simulink model "TVC_3D"  (R2020b)
settings: Solver=VariableStepAuto  StartTime=0.0  StopTime=10.0  RelTol=1e-3
libraries: pid_lib x2, shared6dof x1
settings Model: Creator=mluser  LastModifiedBy=avina

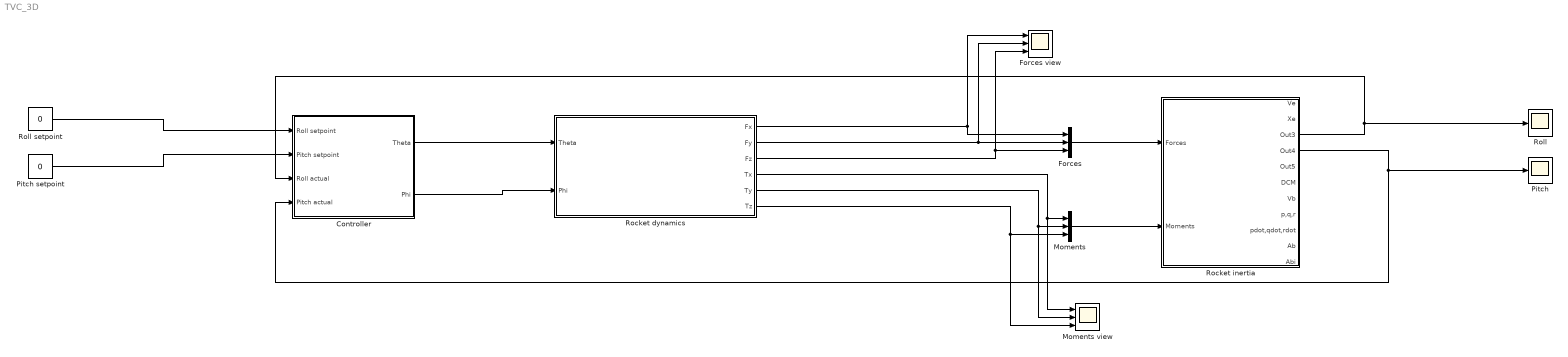
== system TVC_3D ==
  Controller : Subsystem
  Forces : Mux  Inputs=3
  Forces view : Scope  NumInputPorts=3
  Moments : Mux  Inputs=3
  Moments view : Scope  NumInputPorts=3
  Pitch : Scope
  Pitch setpoint : Constant  Value=0
  Rocket dynamics : Subsystem
  Rocket inertia : Subsystem
  Roll : Scope
  Roll setpoint : Constant  Value=0
  wires:
  Roll setpoint/1 -> Controller/1(Roll setpoint)
  Pitch setpoint/1 -> Controller/2(Pitch setpoint)
  Rocket dynamics/4(Tx) -> Moments view/1, Moments/1
  Rocket dynamics/3(Fz) -> Forces/3, Forces view/3
  Rocket dynamics/5(Ty) -> Moments view/2, Moments/2
  Rocket dynamics/1(Fx) -> Forces view/1, Forces/1
  Rocket dynamics/2(Fy) -> Forces view/2, Forces/2
  Rocket dynamics/6(Tz) -> Moments view/3, Moments/3
  Controller/1(Theta) -> Rocket dynamics/1(Theta)
  Controller/2(Phi) -> Rocket dynamics/2(Phi)
  Rocket inertia/4(Out4) -> Controller/4(Pitch actual), Pitch/1
  Rocket inertia/3(Out3) -> Controller/3(Roll actual), Roll/1
  Forces/1 -> Rocket inertia/1(Forces)
  Moments/1 -> Rocket inertia/2(Moments)

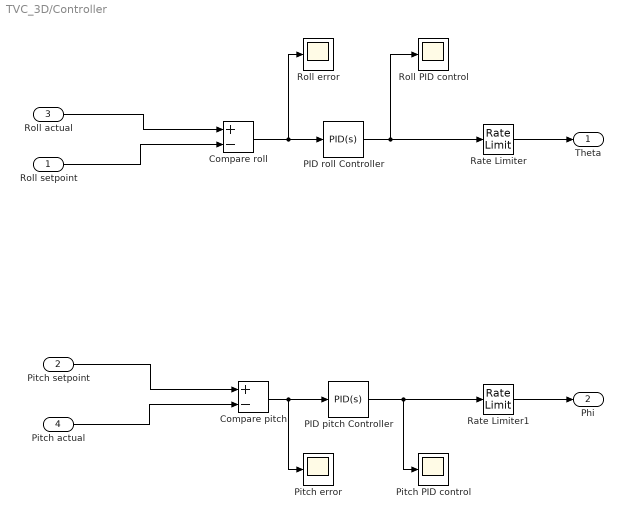
== system TVC_3D/Controller ==
  Roll setpoint : Inport
  Pitch setpoint : Inport  Port=2
  Roll actual : Inport  Port=3
  Pitch actual : Inport  Port=4
  Compare pitch : Sum  Inputs=+-
  Compare roll : Sum  Inputs=+-
  PID pitch Controller : pid_lib/PID Controller  Controller=PID  Form=Parallel  TimeDomain=Continuous-time  UseExternalTs=off  SampleTime=-1  IntegratorMethod=Forward Euler  FilterMethod=Forward Euler  ControllerParametersSource=internal  P=0.2  I=0.00047  D=0.06  UseFilter=on  N=100  TunerSelectOption=Transfer Function Based (PID Tuner App)  InitialConditionSource=internal  InitialConditionForIntegrator=0  InitialConditionForFilter=0  DifferentiatorICPrevScaledInput=0  ExternalReset=none  TrackingMode=off  Kt=1  LimitOutput=on  SatLimitsSource=internal  UpperSaturationLimit=0.349  LowerSaturationLimit=-0.349  LinearizeAsGain=on  AntiWindupMode=none  Kb=1  POutMin=[]  POutMax=[]  IOutMin=[]  IOutMax=[]  DOutMin=[]  DOutMax=[]  NOutMin=[]  NOutMax=[]  SumOutMin=[]  SumOutMax=[]  SaturationOutMin=[]  SaturationOutMax=[]  PParamMin=[]  PParamMax=[]  IParamMin=[]  IParamMax=[]  DParamMin=[]  DParamMax=[]  NParamMin=[]  NParamMax=[]  KbParamMin=[]  KbParamMax=[]  KtParamMin=[]  KtParamMax=[]  KbOutMin=[]  KbOutMax=[]  KtOutMin=[]  KtOutMax=[]  IntegratorOutMin=[]  IntegratorOutMax=[]  FilterOutMin=[]  FilterOutMax=[]  SumI1OutMin=[]  SumI1OutMax=[]  SumI2OutMin=[]  SumI2OutMax=[]  SumI3OutMin=[]  SumI3OutMax=[]  SumI4OutMin=[]  SumI4OutMax=[]  SumDOutMin=[]  SumDOutMax=[]  DifferentiatorOutMin=[]  DifferentiatorOutMax=[]  FilterDiffOutCoefMin=[]  FilterDiffOutCoefMax=[]  ReciprocalOutMin=[]  ReciprocalOutMax=[]  SumDenOutMin=[]  SumDenOutMax=[]  SumNumOutMin=[]  SumNumOutMax=[]  DivideOutMin=[]  DivideOutMax=[]  UdiffTsProdOutMin=[]  UdiffTsProdOutMax=[]  NTsProdOutMin=[]  NTsProdOutMax=[]  UintegralTsProdOutMin=[]  UintegralTsProdOutMax=[]  UngainTsProdOutMin=[]  UngainTsProdOutMax=[]  IntegratorContinuousStateAttributes=''  IntegratorStateMustResolveToSignalObject=off  IntegratorRTWStateStorageClass=Auto  FilterContinuousStateAttributes=''  FilterStateMustResolveToSignalObject=off  FilterRTWStateStorageClass=Auto  ParallelPVariant=InternalParameters  IdealPVariant=Disabled  IVariant=InternalParameters  DVariant=InternalParameters  IntegratorVariant=Continuous  SatVariant=Enabled  AWVariant=Passthrough  PCopyVariant=Disabled  TRVariant=Disabled  FdbkBlocksVariant=Forward  IdealPFdbkVariant=Disabled  SatFdbkVariant=Disabled  DerivativeFilterVariant=ContFilter  NVariant=InternalParameters  NCopyVariant=Disabled  FilterICVariant=InternalICsFilter  IntegratorICVariant=InternalICs  ExternalResetVariant=Disabled  TRSumVariant=Passthrough  SumFdbkVariant=Disabled  SumVariant=Sum_PID  TsampFilterVariant=InternalTs  TsampNgainVariant=Passthrough  TsampIntegralVariant=Passthrough  ExternalSaturationOutDataTypeStr=Inherit: Same as second input
  PID roll Controller : pid_lib/PID Controller  Controller=PID  Form=Parallel  TimeDomain=Continuous-time  UseExternalTs=off  SampleTime=-1  IntegratorMethod=Forward Euler  FilterMethod=Forward Euler  ControllerParametersSource=internal  P=0.2  I=0  D=0.06  UseFilter=on  N=100  TunerSelectOption=Transfer Function Based (PID Tuner App)  InitialConditionSource=internal  InitialConditionForIntegrator=0  InitialConditionForFilter=0  DifferentiatorICPrevScaledInput=0  ExternalReset=none  TrackingMode=off  Kt=1  LimitOutput=on  SatLimitsSource=internal  UpperSaturationLimit=0.349  LowerSaturationLimit=-0.349  LinearizeAsGain=on  AntiWindupMode=none  Kb=1  POutMin=[]  POutMax=[]  IOutMin=[]  IOutMax=[]  DOutMin=[]  DOutMax=[]  NOutMin=[]  NOutMax=[]  SumOutMin=[]  SumOutMax=[]  SaturationOutMin=[]  SaturationOutMax=[]  PParamMin=[]  PParamMax=[]  IParamMin=[]  IParamMax=[]  DParamMin=[]  DParamMax=[]  NParamMin=[]  NParamMax=[]  KbParamMin=[]  KbParamMax=[]  KtParamMin=[]  KtParamMax=[]  KbOutMin=[]  KbOutMax=[]  KtOutMin=[]  KtOutMax=[]  IntegratorOutMin=[]  IntegratorOutMax=[]  FilterOutMin=[]  FilterOutMax=[]  SumI1OutMin=[]  SumI1OutMax=[]  SumI2OutMin=[]  SumI2OutMax=[]  SumI3OutMin=[]  SumI3OutMax=[]  SumI4OutMin=[]  SumI4OutMax=[]  SumDOutMin=[]  SumDOutMax=[]  DifferentiatorOutMin=[]  DifferentiatorOutMax=[]  FilterDiffOutCoefMin=[]  FilterDiffOutCoefMax=[]  ReciprocalOutMin=[]  ReciprocalOutMax=[]  SumDenOutMin=[]  SumDenOutMax=[]  SumNumOutMin=[]  SumNumOutMax=[]  DivideOutMin=[]  DivideOutMax=[]  UdiffTsProdOutMin=[]  UdiffTsProdOutMax=[]  NTsProdOutMin=[]  NTsProdOutMax=[]  UintegralTsProdOutMin=[]  UintegralTsProdOutMax=[]  UngainTsProdOutMin=[]  UngainTsProdOutMax=[]  IntegratorContinuousStateAttributes=''  IntegratorStateMustResolveToSignalObject=off  IntegratorRTWStateStorageClass=Auto  FilterContinuousStateAttributes=''  FilterStateMustResolveToSignalObject=off  FilterRTWStateStorageClass=Auto  ParallelPVariant=InternalParameters  IdealPVariant=Disabled  IVariant=InternalParameters  DVariant=InternalParameters  IntegratorVariant=Continuous  SatVariant=Enabled  AWVariant=Passthrough  PCopyVariant=Disabled  TRVariant=Disabled  FdbkBlocksVariant=Forward  IdealPFdbkVariant=Disabled  SatFdbkVariant=Disabled  DerivativeFilterVariant=ContFilter  NVariant=InternalParameters  NCopyVariant=Disabled  FilterICVariant=InternalICsFilter  IntegratorICVariant=InternalICs  ExternalResetVariant=Disabled  TRSumVariant=Passthrough  SumFdbkVariant=Disabled  SumVariant=Sum_PID  TsampFilterVariant=InternalTs  TsampNgainVariant=Passthrough  TsampIntegralVariant=Passthrough  ExternalSaturationOutDataTypeStr=Inherit: Same as second input
  Pitch PID control : Scope
  Pitch error : Scope
  Rate Limiter : RateLimiter  RisingSlewLimit=500  FallingSlewLimit=-500  SampleTimeMode=inherited
  Rate Limiter1 : RateLimiter  RisingSlewLimit=500  FallingSlewLimit=-500  SampleTimeMode=inherited
  Roll PID control : Scope
  Roll error : Scope
  Theta : Outport
  Phi : Outport  Port=2
  wires:
  PID pitch Controller/1 -> Pitch PID control/1, Rate Limiter1/1
  PID roll Controller/1 -> Roll PID control/1, Rate Limiter/1
  Roll setpoint/1 -> Compare roll/2
  Compare roll/1 -> Roll error/1, PID roll Controller/1
  Pitch actual/1 -> Compare pitch/2
  Compare pitch/1 -> Pitch error/1, PID pitch Controller/1
  Roll actual/1 -> Compare roll/1
  Pitch setpoint/1 -> Compare pitch/1
  Rate Limiter/1 -> Theta/1
  Rate Limiter1/1 -> Phi/1

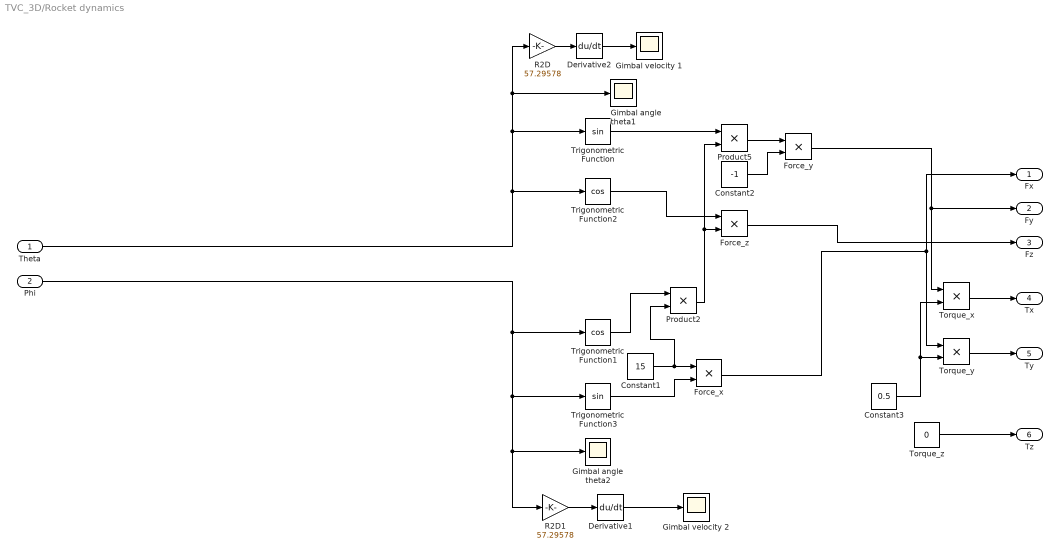
== system TVC_3D/Rocket dynamics ==
  Theta : Inport
  Phi : Inport  Port=2
  Constant1 : Constant  Value=15
  Constant2 : Constant  Value=-1
  Constant3 : Constant  Value=0.5
  Derivative1 : Derivative
  Derivative2 : Derivative
  Force_x : Product
  Force_y : Product
  Force_z : Product
  Gimbal angle theta1 : Scope
  Gimbal angle theta2 : Scope
  Gimbal velocity 1 : Scope
  Gimbal velocity 2 : Scope
  Product2 : Product
  Product5 : Product
  R2D : Gain  Gain=57.29578
  R2D1 : Gain  Gain=57.29578
  Torque_x : Product
  Torque_y : Product
  Torque_z : Constant  Value=0
  Trigonometric Function : Trigonometry
  Trigonometric Function1 : Trigonometry  Operator=cos
  Trigonometric Function2 : Trigonometry  Operator=cos
  Trigonometric Function3 : Trigonometry
  Fx : Outport
  Fy : Outport  Port=2
  Fz : Outport  Port=3
  Tx : Outport  Port=4
  Ty : Outport  Port=5
  Tz : Outport  Port=6
  wires:
  Product2/1 -> Product5/2, Force_z/2
  Derivative2/1 -> Gimbal velocity 1/1
  Theta/1 -> R2D/1, Gimbal angle theta1/1, Trigonometric Function/1, Trigonometric Function2/1
  Force_x/1 -> Fx/1, Torque_y/1
  Constant1/1 -> Force_x/1, Product2/2
  Trigonometric Function2/1 -> Force_z/1
  Phi/1 -> R2D1/1, Gimbal angle theta2/1, Trigonometric Function3/1, Trigonometric Function1/1
  Torque_x/1 -> Tx/1
  Torque_y/1 -> Ty/1
  Trigonometric Function3/1 -> Force_x/2
  Constant3/1 -> Torque_x/2, Torque_y/2
  Force_z/1 -> Fz/1
  Trigonometric Function/1 -> Product5/1
  Product5/1 -> Force_y/1
  Constant2/1 -> Force_y/2
  Trigonometric Function1/1 -> Product2/1
  Force_y/1 -> Torque_x/1, Fy/1
  Derivative1/1 -> Gimbal velocity 2/1
  R2D/1 -> Derivative2/1
  R2D1/1 -> Derivative1/1
  Torque_z/1 -> Tz/1

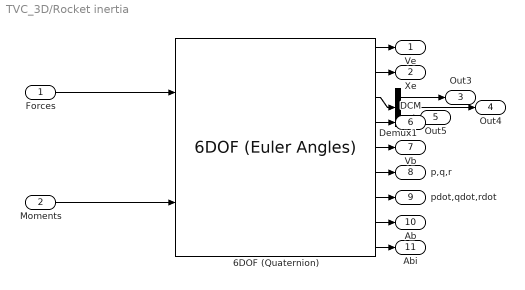
== system TVC_3D/Rocket inertia ==
  Forces : Inport
  Moments : Inport  Port=2
  6DOF (Quaternion) : shared6dof/6DOF (Euler Angles)  units=Metric (MKS)  mtype=Fixed  rep=Euler Angles  xme_0=[0 0 0]  Vm_0=[0 0 0]  eul_0=[0.698 0.0837 0]  pm_0=[0 0 0]  mass_0=1.0  mass_e=0.5  mass_f=2.0  inertia="[0.08583 0 0;  0 0.08583 0; 0 0 0.00083]"  inertia_e=eye(3)  inertia_f=2*eye(3)  k_quat=1.0  vre_flag=on  abi_flag=on  aMode=0  xme_statename=''  Vm_statename=''  eul_statename=''  quat_statename=''  pm_statename=''  mass_statename=''
      settings: SourceProductBaseCode=AE,PW,MT,UV,VE,VP
  Demux1 : Demux  Outputs=3
  Ve : Outport
  Xe : Outport  Port=2
  Out3 : Outport  Port=3
  Out4 : Outport  Port=4
  Out5 : Outport  Port=5
  DCM : Outport  Port=6
  Vb : Outport  Port=7
  p,q,r : Outport  Port=8
  pdot,qdot,rdot : Outport  Port=9
  Ab : Outport  Port=10
  Abi : Outport  Port=11
  wires:
  6DOF (Quaternion)/4 -> DCM/1
  Demux1/1 -> Out3/1
  Moments/1 -> 6DOF (Quaternion)/2
  6DOF (Quaternion)/8 -> Ab/1
  6DOF (Quaternion)/5 -> Vb/1
  6DOF (Quaternion)/3 -> Demux1/1
  Forces/1 -> 6DOF (Quaternion)/1
  Demux1/2 -> Out4/1
  6DOF (Quaternion)/1 -> Ve/1
  Demux1/3 -> Out5/1
  6DOF (Quaternion)/2 -> Xe/1
  6DOF (Quaternion)/7 -> pdot,qdot,rdot/1
  6DOF (Quaternion)/6 -> p,q,r/1
  6DOF (Quaternion)/9 -> Abi/1
